simulink model "aMPC_for_embedded_with_subsystem"  (R2019a)
settings: Solver=ode1  StartTime=0.0  StopTime=15  FixedStep=0.01  RelTol=1e-3  EnableMultiTasking=on
libraries: simulink x1, mpclib x1
settings Model: Creator=alexh  LastModifiedBy=alexh
settings SolverCC: PositivePriorityOrder=on  AutoInsertRateTranBlk=on
settings OptimizationCC: DefaultParameterBehavior=Inlined  UseDivisionForNetSlopeComputation=on  GainParamInheritBuiltInType=on  UseFloatMulNetSlope=on  InlineInvariantSignals=on  PassReuseOutputArgsAs=Individual arguments  ZeroExternalMemoryAtStartup=off  ZeroInternalMemoryAtStartup=off  NoFixptDivByZeroProtection=on  EfficientFloat2IntCast=on  LifeSpan=1  MaxStackSize=64  OptimizeBlockOrder=speed  DifferentSizesBufferReuse=on
settings DebuggingCC: ParameterTunabilityLossMsg=error
settings HardwareCC: ProdBitPerPointer=32  ProdBitPerSizeT=32  ProdBitPerPtrDiffT=32  ProdLargestAtomicInteger=Long  ProdWordSize=32  ProdHWDeviceType=ARM Compatible->ARM 10
settings SFSimCC: MATLABDynamicMemAlloc=off
settings RTWCC: SystemTargetFile=ert.tlc  TemplateMakefile=ert_default_tmf  GenerateReport=on  Toolchain=GNU GCC Raspberry Pi  BuildConfiguration=Debug  IncludeHyperlinkInReport=on  LaunchReport=on  GenerateTraceInfo=on  GenerateTraceReport=on  GenerateTraceReportSl=on  GenerateTraceReportSf=on  GenerateTraceReportEml=on  GenerateCodeMetricsReport=on
settings CodeAppCC: ForceParamTrailComments=on  IgnoreCustomStorageClasses=off  OperatorAnnotations=on  SimulinkDataObjDesc=on  SFDataObjDesc=on  CustomSymbolStrGlobalVar=rt$N$M  CustomSymbolStrType=$N$M  CustomSymbolStrFcn=$N$M$F  CustomSymbolStrMacro=$N$M  InsertBlockDesc=on
settings ERTTargetCC: TargetLangStandard=C99 (ISO)  IncludeMdlTerminateFcn=off  CombineSignalStateStructs=on  SupportAbsoluteTime=off  SupportComplex=off  SupportContinuousTime=on  SupportNonInlinedSFcns=on  InlinedParameterPlacement=NonHierarchical  ERTCustomFileTemplate=example_file_process.tlc  ERTFilePackagingFormat=CompactWithDataFile

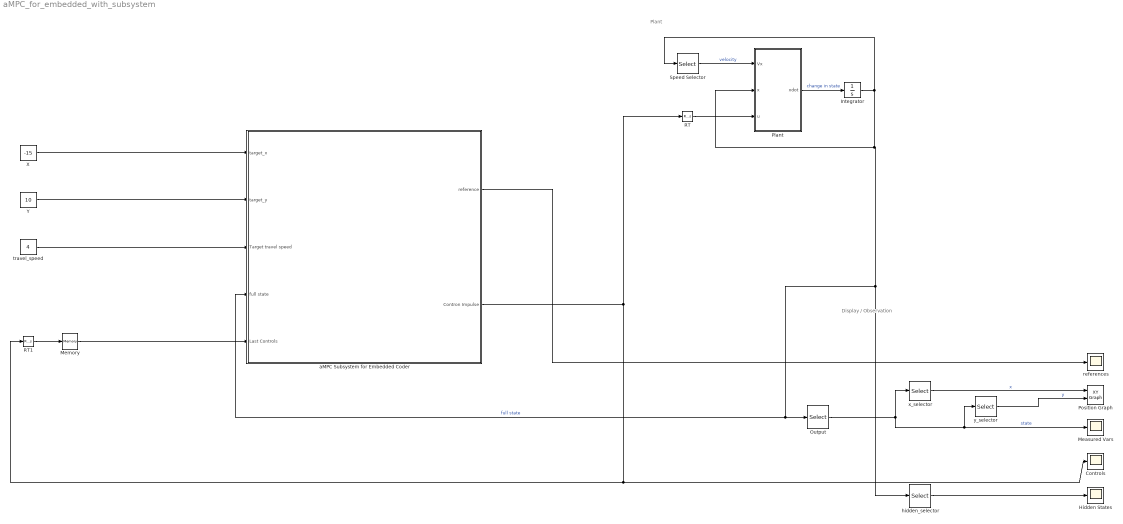
== system aMPC_for_embedded_with_subsystem ==
  note: Plant
  note: Display / Observation
  Controls : Scope
  Hidden States : Scope
  Integrator : Integrator
  Measured Vars : Scope
  Memory : Memory
  Output : Selector  InputPortWidth=6  IndexOptions=Index vector (dialog)  Indices=[1, 2, 3, 6]  OutputSizes=1
  "Plant " : MATLAB Function  TreatAsAtomicUnit=on
  Position Graph : simulink/Sinks/XY Graph  xmin=-15  xmax=15  ymin=-15  ymax=15  st=-1
  RT : RateTransition  OutPortSampleTime=0.01
  RT1 : RateTransition  OutPortSampleTime=0.01
  Speed Selector : Selector  InputPortWidth=6  IndexOptions=Index vector (dialog)  Indices=[6]  OutputSizes=1
  X : Constant  Value=-15
  Y : Constant  Value=10
  aMPC Subsystem for Embedded Coder : Subsystem
  hidden_selector : Selector  InputPortWidth=6  IndexOptions=Index vector (dialog)  Indices=[4, 5]  OutputSizes=1
  references : Scope
  travel_speed : Constant  Value=4
  x_selector : Selector  InputPortWidth=4  IndexOptions=Index vector (dialog)  Indices=[1]  OutputSizes=1
  y_selector : Selector  InputPortWidth=4  IndexOptions=Index vector (dialog)  Indices=[2]  OutputSizes=1
  wires:
  "Plant "/1(xdot) -> Integrator/1  "change in state"
  Output/1 -> x_selector/1, Measured Vars/1, y_selector/1  "state"
  x_selector/1 -> Position Graph/1  "x"
  y_selector/1 -> Position Graph/2  "y"
  hidden_selector/1 -> Hidden States/1
  Integrator/1 -> "Plant "/2(x), hidden_selector/1, aMPC Subsystem for Embedded Coder/4(full state), Output/1, Speed Selector/1  "full state"
  Speed Selector/1 -> "Plant "/1(Vx)  "velocity"
  RT/1 -> "Plant "/3(u)
  RT1/1 -> Memory/1
  aMPC Subsystem for Embedded Coder/2(Contron Impulse) -> RT/1, Controls/1, RT1/1
  X/1 -> aMPC Subsystem for Embedded Coder/1(target_x)
  Y/1 -> aMPC Subsystem for Embedded Coder/2(target_y)
  travel_speed/1 -> aMPC Subsystem for Embedded Coder/3(Target travel speed)
  Memory/1 -> aMPC Subsystem for Embedded Coder/5(Last Controls)
  aMPC Subsystem for Embedded Coder/1(reference) -> references/1

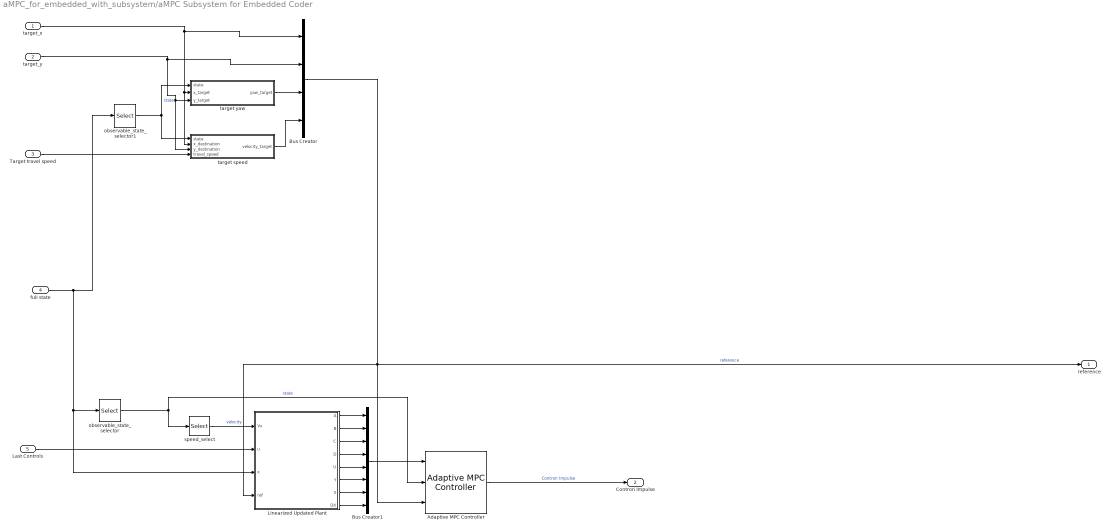
== system aMPC_for_embedded_with_subsystem/aMPC Subsystem for Embedded Coder ==
  target_x : Inport
  target_y : Inport  Port=2
  Target travel speed : Inport  Port=3
  full state : Inport  Port=4
  Last Controls : Inport  Port=5
  Adaptive MPC Controller : mpclib/Adaptive MPC Controller  SCDEnableBlockLinearizationSpecification=on  mpcobj=bycicle_mpc  enable_value=0  updateMPCinCallerWorkspace=on  md_inport=off  mv_inport=off  uref_inport=off  return_cost=off  return_mvseq=off  return_qpstatus=off  return_xseq=off  return_state=off  return_ovseq=off  state_inport=off  isltv_plant=off  umin_inport=off  umax_inport=off  ymin_inport=off  ymax_inport=off  cc_inport=off  ywt_inport=off  uwt_inport=off  duwt_inport=off  rhoeps_inport=off  pm_inport=off  MaximumP=10  HorizonChoice=FixedHorizon  BlockDataType=double  SampleTimeInherited=off  switch_inport=off
      settings: SourceProductName=MATLAB Runtime - Model Predictive Control Toolbox Addin  SourceProductBaseCode=Missing
  Bus Creator : BusCreator  Inputs=4
  Bus Creator1 : BusCreator  Inputs=8
  Linearized Updated Plant : MATLAB Function  TreatAsAtomicUnit=on
  observable_state_selector : Selector  InputPortWidth=6  IndexOptions=Index vector (dialog)  Indices=[1, 2, 3, 6]  OutputSizes=1
  observable_state_selector1 : Selector  InputPortWidth=6  IndexOptions=Index vector (dialog)  Indices=[1, 2, 3, 6]  OutputSizes=1
  speed_select : Selector  InputPortWidth=4  IndexOptions=Index vector (dialog)  Indices=[4]  OutputSizes=1
  target speed : MATLAB Function  TreatAsAtomicUnit=on
  target yaw : MATLAB Function  TreatAsAtomicUnit=on
  reference : Outport
  Contron Impulse : Outport  Port=2
  wires:
  full state/1 -> Linearized Updated Plant/3(x), observable_state_selector/1, observable_state_selector1/1
  Linearized Updated Plant/7(X) -> Bus Creator1/7
  Linearized Updated Plant/5(U) -> Bus Creator1/5
  Linearized Updated Plant/1(A) -> Bus Creator1/1
  target speed/1(velocity_target) -> Bus Creator/4
  Linearized Updated Plant/3(C) -> Bus Creator1/3
  Bus Creator1/1 -> Adaptive MPC Controller/1
  Linearized Updated Plant/4(D) -> Bus Creator1/4
  target_x/1 -> target speed/2(x_destination), target yaw/2(x_target), Bus Creator/1
  speed_select/1 -> Linearized Updated Plant/1(Vx)  "velocity"
  Linearized Updated Plant/2(B) -> Bus Creator1/2
  Bus Creator/1 -> reference/1, Adaptive MPC Controller/3, Linearized Updated Plant/4(ref)  "reference"
  Adaptive MPC Controller/1 -> Contron Impulse/1  "Contron Impulse"
  Linearized Updated Plant/8(DX) -> Bus Creator1/8
  Linearized Updated Plant/6(Y) -> Bus Creator1/6
  target_y/1 -> Bus Creator/2, target speed/3(y_destination), target yaw/3(y_target)
  target yaw/1(yaw_target) -> Bus Creator/3
  observable_state_selector/1 -> Adaptive MPC Controller/2, speed_select/1  "state"
  observable_state_selector1/1 -> target speed/1(state), target yaw/1(state)  "state"
  Last Controls/1 -> Linearized Updated Plant/2(u)
  Target travel speed/1 -> target speed/4(travel_speed)

== matlab function aMPC_for_embedded_with_subsystem/aMPC Subsystem for Embedded Coder/Linearized Updated Plant ==
  data: Vx input; u input; A output; x input; B output; C output; D output; U output; Y output; X output; DX output; ref input
function [A,B,C,D,U,Y,X,DX] = fcn(Vx,u,x, ref)
% Sample time
Ts = 0.1;

% Model parameters
m = 1575;
iz = 2875;
lf = 1.2;
lr = 1.6;
cf = 19000;
cr = 33000;

if (Vx<1)
       Vx = 1;
end

% we have to tweak the system a bit to make it realize altering the 
% speed can do something for reaching the destination
if (x(2)<ref(2))
    speed_influence = 0.1;
else
    speed_influence = -0.1;
end

% Continuous-time model
Ac = [0, 0, -Vx, 0, -1, Vx;
       0, 0, Vx, 0, 1, speed_influence;
       0, 0, 0, 1, 0, 0;
       0, 0, 0, -(2*cf*lf^2+2*cr*lr^2)/iz/Vx, -(2*cf*lf-2*cr*lr)/iz/Vx, 0;
       0, 0, 0,  -Vx-(2*cf*lf-2*cr*lr)/m/Vx, -(2*cf+2*cr)/m/Vx, 0;
       0, 0, 0, 0, 0, -.1];
   
 Bc = [0, 0, 0, 2*cf*lf/iz, 2*cf/m, 0;
        0, 0, 0, 0, 0, 1]';
 
 % Position, Yaw, Speed
 Cc = [1, 0, 0, 0, 0, 0;
        0, 1, 0, 0, 0, 0;
        0, 0, 1, 0, 0, 0;
        0, 0, 0, 0, 0, 1];
    
 Dc = zeros(4, 2);

% Generate discrete-time model
nx = size(Ac,1);
nu = size(Bc,2);
M = expm([[Ac Bc]*Ts; zeros(nu,nx+nu)]);
A = M(1:nx,1:nx);
B = M(1:nx,nx+1:nx+nu);
C = Cc;
D = Dc;

% Nominal conditions for discrete-time plant
X = x';
U = u';
Y = (C*x + D*u)';
DX = (A*x+B*u-x)';      % did this fix, might be wrong

== matlab function aMPC_for_embedded_with_subsystem/Plant  ==
  data: Vx input; x input; u input; xdot output
function xdot = fcn(Vx,x,u)

if (Vx<1)
    Vx=1;
end

% Model parameters
m = 1575;
iz = 2875;
lf = 1.2;
lr = 1.6;
cf = 19000;
cr = 33000;

sin_yaw = sin(x(3));
cos_yaw = cos(x(3));


% Continuous-time model
% Continuous-time model
Ac = [0, 0, 0, 0, 0, cos_yaw;
       0, 0, 0, 0, 0, sin_yaw;
       0, 0, 0, 1, 0, 0;
       0, 0, 0, -(2*cf*lf^2+2*cr*lr^2)/iz/Vx, -(2*cf*lf-2*cr*lr)/iz/Vx, 0;
       0, 0, 0,  -Vx-(2*cf*lf-2*cr*lr)/m/Vx, -(2*cf+2*cr)/m/Vx, 0;
       0, 0, 0, 0, 0, -.1];
   
 Bc = [0, 0, 0, 2*cf*lf/iz, 2*cf/m, 0;
        0, 0, 0, 0, 0, 1]';

xdot = Ac*x + Bc*u;

== matlab function aMPC_for_embedded_with_subsystem/aMPC Subsystem for Embedded Coder/target yaw ==
  data: state input; yaw_target output; x_target input; y_target input
function yaw_target = fcn(state, x_target, y_target)

% Rearange data
position = [state(1) state(2)];
position_target = [x_target, y_target]';
x = state(1);
y = state(2);
yaw = state(3);

% Calculate target yaw
yaw_target = atan((abs(y) - abs(y_target)) / (abs(x) - abs(x_target)));
if x - x_target > 0 && y - y_target < 0         % 2nd q
    yaw_target = pi - yaw_target;
elseif x - x_target > 0 && y - y_target > 0     % 3rd q
    yaw_target = -pi + yaw_target;
elseif x - x_target < 0 && y - y_target > 0     % 4th q
    yaw_target = -yaw_target;
end

% Adjust so we actually take shortest doff
yaw_diff = acos((position * position_target) / (norm(position) * norm(position_target)));

%if ((yaw + yaw_diff) > pi) && (yaw > yaw_target)
%    yaw_target = yaw_target + 2*pi;
%elseif((yaw - yaw_diff) < -pi) && (yaw < yaw_target)
%    yaw_target = yaw_target - 2*pi;
%end

if yaw_diff < pi
    if yaw_target < 0 && yaw > 0
        yaw_target = yaw_target + 2*pi;
    end
    if yaw_target > 0 && yaw < 0
        yaw_target = yaw_target - 2*pi;
    end    
end

== matlab function aMPC_for_embedded_with_subsystem/aMPC Subsystem for Embedded Coder/target speed ==
  data: state input; velocity_target output; x_destination input; y_destination input; travel_speed input
function velocity_target = fcn(state, x_destination, y_destination, travel_speed)

% Rearange data
position = [state(1) state(2)];
position_target = [x_destination, y_destination];

% Calculate delta position
delta_position = position - position_target;

distance_to_travel = norm(delta_position);

velocity_target = min(travel_speed, distance_to_travel/2);
